simulink model "MG1"  (R2020b)
settings: Solver=VariableStepAuto  StartTime=0.0  StopTime=TFinal  FixedStep=0.01  RelTol=1e-3
undefined symbols (not defined in the file or in its folder): B, G, n, Nodes
libraries: simulink x1
settings Model: Creator=tian  LastModifiedBy=tian

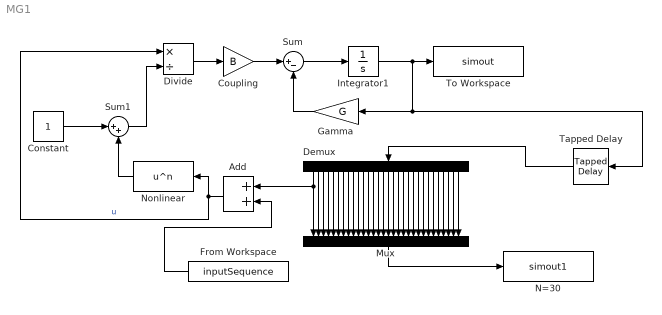
== system MG1 ==
  Add : Sum
  Constant : Constant
  Coupling : Gain  Gain=B
  Demux : Demux  Outputs=30
  Divide : Product  Inputs=*/
  From Workspace : FromWorkspace  VariableName=inputSequence
  Gamma : Gain  Gain=G
  Integrator1 : Integrator
  Mux : Mux  Inputs=30
  N=30 : ToWorkspace  VariableName=simout1  SampleTime=-1
  Nonlinear : Fcn  Expr=u^n
  Sum : Sum  Inputs=|+-
  Sum1 : Sum  Inputs=|++
  Tapped Delay : simulink/Discrete/Tapped Delay  vinit=0.0  samptime=TDelay  NumDelays=Nodes  DelayOrder=Oldest  includeCurrent=off
  To Workspace : ToWorkspace  VariableName=simout  SampleTime=-1
      settings: Save2DSignal=2-D array (concatenate along first dimension)
  wires:
  Coupling/1 -> Sum/1
  Nonlinear/1 -> Sum1/2
  Gamma/1 -> Sum/2
  Sum1/1 -> Divide/2
  Constant/1 -> Sum1/1
  Add/1 -> Nonlinear/1, Divide/1  "u"
  Integrator1/1 -> To Workspace/1, Tapped Delay/1, Gamma/1
  Divide/1 -> Coupling/1
  Sum/1 -> Integrator1/1
  Mux/1 -> N=30/1
  Demux/1 -> Mux/1, Add/1
  Demux/2 -> Mux/2
  Demux/3 -> Mux/3
  Demux/5 -> Mux/5
  Demux/4 -> Mux/4
  Demux/6 -> Mux/6
  Demux/7 -> Mux/7
  Demux/8 -> Mux/8
  Demux/10 -> Mux/10
  Demux/9 -> Mux/9
  Demux/11 -> Mux/11
  Demux/13 -> Mux/13
  Demux/12 -> Mux/12
  Demux/14 -> Mux/14
  Demux/15 -> Mux/15
  Demux/16 -> Mux/16
  Demux/17 -> Mux/17
  Demux/18 -> Mux/18
  Demux/19 -> Mux/19
  Demux/20 -> Mux/20
  Demux/21 -> Mux/21
  Demux/22 -> Mux/22
  Demux/23 -> Mux/23
  Demux/24 -> Mux/24
  Demux/25 -> Mux/25
  Demux/27 -> Mux/27
  Demux/28 -> Mux/28
  Demux/29 -> Mux/29
  Demux/30 -> Mux/30
  Demux/26 -> Mux/26
  Tapped Delay/1 -> Demux/1
  From Workspace/1 -> Add/2
